simulink model "observador_simulink"  (R2017b)
settings: Solver=VariableStepAuto  StartTime=0.0  StopTime=30  FixedStep=0.00527  RelTol=1e-3
values from neighbouring files (symbols this model uses):
  A = [-b/J K/J; -K/L R/L]    [distance.m]    (also in kp_script.m = [0 -1/(R*CS); 0 0]; model_params.m; observador_script.m)
  Adps = Adp    [observador_script.m]
  B = [0;1/L]    [distance.m]    (also in kp_script.m = [0 ; -1/(R*CS)]; model_params.m; observador_script.m)
  Bdps = Bdp    [observador_script.m]
  C = [1,0]    [distance.m]    (also in kp_script.m = [1 0]; model_params.m; observador_script.m)
  Cpssensor = [1 0 0 0 0]    [observador_script.m]
  D = 0    [distance.m]    (also in kp_script.m; model_params.m; observador_script.m)
  kd = acker(Ad, Bd, polsd)    [kp_script.m]    (also in observador_script.m)
  Ldps = (acker(Adps',Cpssensor',[polsod(1) polsod(2) 0.9 0.9+0.1i 0.9-0.1i]))'    [observador_script.m]
  Nu = N(3)    [kp_script.m]    (also in observador_script.m)
  Nx = N(1:2)    [kp_script.m]    (also in observador_script.m)
settings Model: Creator=guillem.casado  LastModifiedBy=guillem.casado

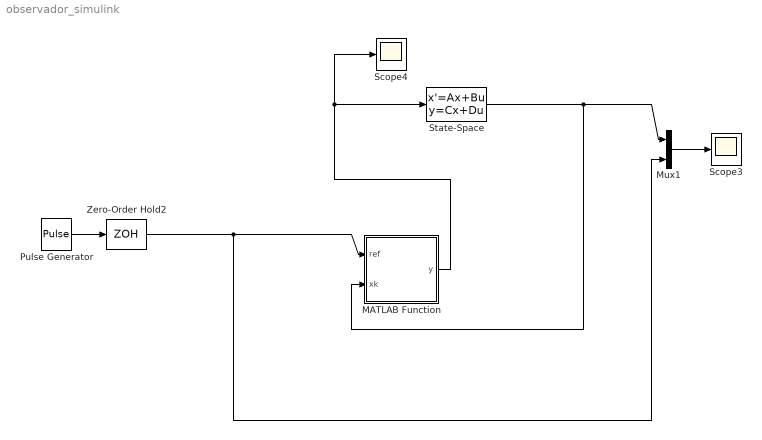
== system observador_simulink ==
  MATLAB Function : MATLAB Function  TreatAsAtomicUnit=on
  Mux1 : Mux  Inputs=2
  Pulse Generator : DiscretePulseGenerator  PulseType=Time based  Amplitude=50  PulseWidth=50
  Scope3 : Scope
  Scope4 : Scope
  State-Space : StateSpace  A=A  B=B  C=C  D=D  InitialCondition=[0,0]
  Zero-Order Hold2 : ZeroOrderHold  SampleTime=0.05
  wires:
  Pulse Generator/1 -> Zero-Order Hold2/1
  Zero-Order Hold2/1 -> Mux1/2, MATLAB Function/1(ref)
  MATLAB Function/1(y) -> Scope4/1, State-Space/1
  State-Space/1 -> Mux1/1, MATLAB Function/2(xk)
  Mux1/1 -> Scope3/1

== matlab function observador_simulink/MATLAB Function ==
  settings: updateMethod=DISCRETE  sampleTime=h
  data: ref input size=1; y output size=1; Nx parameter size=2; Nu parameter size=1; kd parameter size=2; Adps parameter size=[5 5]; Bdps parameter size=5; Cpssensor parameter size=5; Ldps parameter size=5; xk input size=1
function y = fcn(ref,Nx, Nu, kd, Adps, Bdps, Cpssensor, Ldps, xk)
persistent xek
if isempty(xek)
    xek=[0;0;0;0;0];
end

uk=(ref*Nu)+(-kd(1)*(xek(1)-Nx(1)*ref)-kd(2)*(xek(2)-Nx(2)*ref)-xek(3)-xek(4)-xek(5));

xek1=[0;0;0;0;0];
xek1(1)=(uk*Bdps(1))+(xk-(xek(1)*Cpssensor(1)+xek(2)*Cpssensor(2)+xek(3)*Cpssensor(3)+Cpssensor(4)*xek(4)+xek(5)*Cpssensor(5)))*Ldps(1)+(xek(1)*Adps(1,1)+xek(2)*Adps(1,2)+xek(3)*Adps(1,3)+xek(4)*Adps(1,4)++xek(5)*Adps(1,5));
xek1(2)=(uk*Bdps(2))+(xk-(xek(1)*Cpssensor(1)+xek(2)*Cpssensor(2)+xek(3)*Cpssensor(3)+Cpssensor(4)*xek(4)+xek(5)*Cpssensor(5)))*Ldps(2)+(xek(1)*Adps(2,1)+xek(2)*Adps(2,2)+xek(3)*Adps(2,3)+xek(4)*Adps(2,4)++xek(5)*Adps(2,5));
xek1(3)=(uk*Bdps(3))+(xk-(xek(1)*Cpssensor(1)+xek(2)*Cpssensor(2)+xek(3)*Cpssensor(3)+Cpssensor(4)*xek(4)+xek(5)*Cpssensor(5)))*Ldps(3)+(xek(1)*Adps(3,1)+xek(2)*Adps(3,2)+xek(3)*Adps(3,3)+xek(4)*Adps(3,4)++xek(5)*Adps(3,5));
xek1(4)=(uk*Bdps(4))+(xk-(xek(1)*Cpssensor(1)+xek(2)*Cpssensor(2)+xek(3)*Cpssensor(3)+Cpssensor(4)*xek(4)+xek(5)*Cpssensor(5)))*Ldps(4)+(xek(1)*Adps(4,1)+xek(2)*Adps(4,2)+xek(3)*Adps(4,3)+xek(4)*Adps(4,4)++xek(5)*Adps(4,5));
xek1(5)=(uk*Bdps(5))+(xk-(xek(1)*Cpssensor(1)+xek(2)*Cpssensor(2)+xek(3)*Cpssensor(3)+Cpssensor(4)*xek(4)+xek(5)*Cpssensor(5)))*Ldps(5)+(xek(1)*Adps(5,1)+xek(2)*Adps(5,2)+xek(3)*Adps(5,3)+xek(4)*Adps(5,4)++xek(5)*Adps(5,5));
xek(1)=xek1(1);
xek(2)=xek1(2);
xek(3)=xek1(3);
xek(4)=xek1(4);
xek(5)=xek1(5);

y = uk;
